simulink model "test_animation"  (R2021a)
settings: Solver=VariableStepAuto  StartTime=0.0  StopTime=inf  RelTol=1e-3
libraries: simulink x1, vrlib x1
settings Model: Creator=kbhar  LastModifiedBy=kbhar

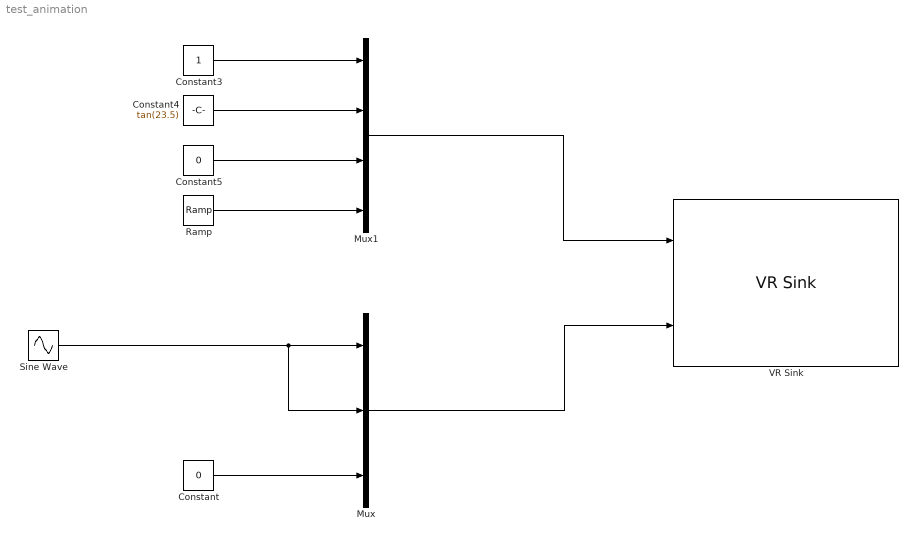
== system test_animation ==
  Constant : Constant  Value=0
  Constant3 : Constant
  Constant4 : Constant  Value=tan(23.5)
  Constant5 : Constant  Value=0
  Mux : Mux  Inputs=3
  Mux1 : Mux
  Ramp : simulink/Sources/Ramp  slope=0.05  start=0  InitialOutput=0
  Sine Wave : Sin  Frequency=0.01  SampleTime=0
  VR Sink : vrlib/VR Sink  InstantiateOnLoad=on  SampleTime=0.1  ViewEnable=on  RemoteChange=off  RemoteView=off  FieldsWritten=theball.rotation.4.1.1.double#theball.translation.3.1.1.double  WorldFileName=C:\Bharat\College\Projects\Arm Control\Files\test_animation.wrl  AutoView=off  VideoDimensions=[]  AllowVariableSize=off
  wires:
  Constant/1 -> Mux/3
  Sine Wave/1 -> Mux/2, Mux/1
  Mux/1 -> VR Sink/2
  Mux1/1 -> VR Sink/1
  Constant4/1 -> Mux1/2
  Constant5/1 -> Mux1/3
  Constant3/1 -> Mux1/1
  Ramp/1 -> Mux1/4
